simulink model "MAIN_simulation"  (R2021b)
settings: Solver=VariableStepAuto  StartTime=0.0  StopTime=10.0  RelTol=1e-3
values from neighbouring files (symbols this model uses):
  N = uint8(10)    [ParamSetup.m]
undefined symbols (not defined in the file or in its folder): Ankle, Hip, Knee, Left, Right, smiData, X, Y, Z
libraries: sm_lib x40, nesl_utility x15
(part 1 of 2)
settings Model: DataDictionary=ExoskeletonParameters.sldd  Creator=user  LastModifiedBy=khoi
settings SolverCC: AlgebraicLoopSolver=LineSearch
settings DebuggingCC: SFMachineParentedDataDiag=warning
settings ModelReferenceCC: EnableParallelModelReferenceBuilds=on  ModelReferenceMinAlgLoopOccurrences=on

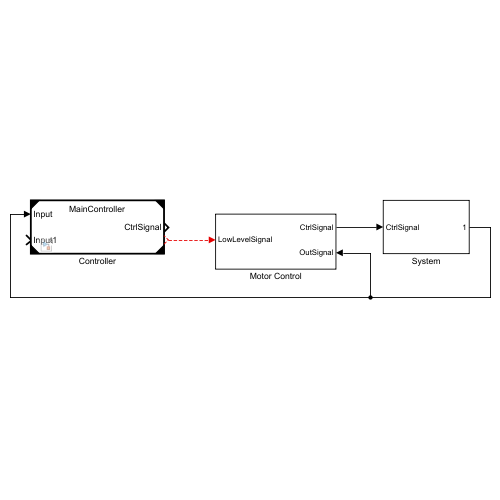
[thumbnail: Simulink's stored preview of the top-level diagram]
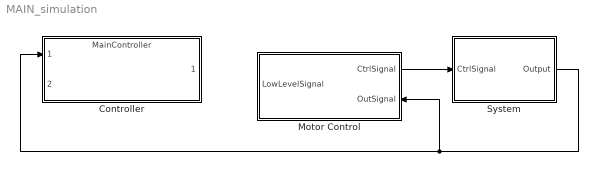
== system MAIN_simulation ==
  Controller : ModelReference  ModelNameDialog=MainController.slx  ModelReferenceVersion=1.32
  Motor Control : Subsystem
      settings: PortSchema="{\"entries\":[{\"content\":{\"sides\":[{\"content\":{\"connectorIds\":[\"In1\"]},\"type\":\"ConnectorPlacement.EquallySpacedRectSide\",\"uuid\":\"f726c4a5-dcc4-4232-8342-e270c8d2deba\"},{\"content\":{\"connectorIds\":[\"Out1\",\"In2\"],\"side\":\"RIGHT\"},\"type\":\"ConnectorPlacement.EquallySpacedRectSide\",\"uuid\":\"fdc8a78d-4edd-4abb-a00a-5ed0e9622b88\"},{\"content\":{\"connectorIds\":[],\"side\":\"TOP\"},\"type\":\"ConnectorPlacement.EquallySpacedRectSide\",\"uuid\":\"7577593d-02f9-4726-9a31-f3a7037643a8\"}]},\"type\":\"ConnectorPlacement.EquallySpacedConnector\",\"uuid\":\"d04c894f-3616-4ed1-83ff-a42822506ca7\"}],\"packageUris\":[\"http://schema.mathworks.com/mf0/Connector/19700101\"],\"version\":\"1.0\"}"
  System : Subsystem
  wires:
  System/1(Output) -> Controller/1, Motor Control/2(OutSignal)
  Motor Control/1(CtrlSignal) -> System/1(CtrlSignal)
  ? -> Motor Control/1(LowLevelSignal)

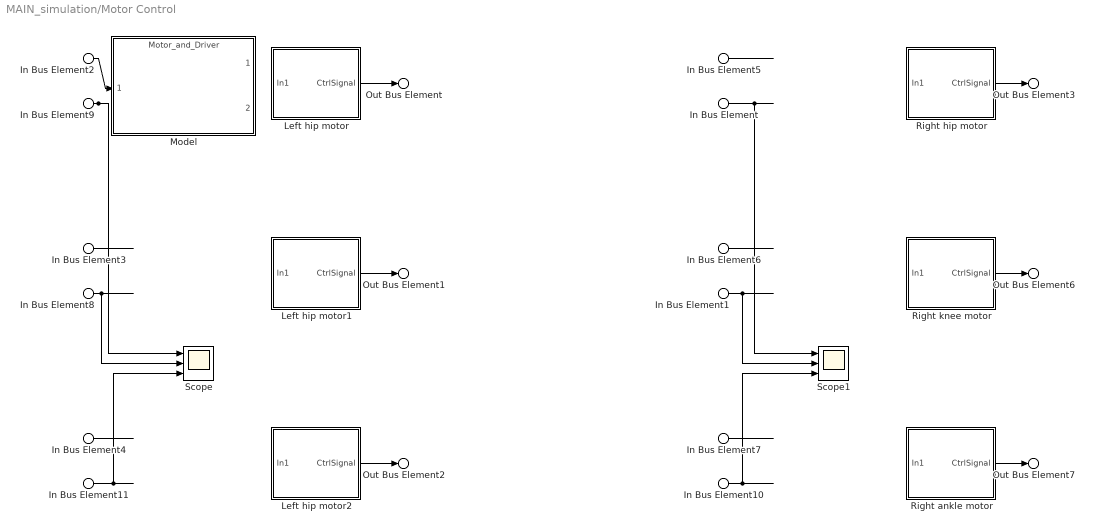
== system MAIN_simulation/Motor Control ==
  In Bus Element2 : Inport  PortName=LowLevelSignal  Element=Left.Hip.Angle
  In Bus Element3 : Inport  PortName=LowLevelSignal  Element=Left.Knee.Angle
  In Bus Element4 : Inport  PortName=LowLevelSignal  Element=Left.Ankle.Angle
  In Bus Element5 : Inport  PortName=LowLevelSignal  Element=Right.Hip.Angle
  In Bus Element6 : Inport  PortName=LowLevelSignal  Element=Right.Knee.Angle
  In Bus Element7 : Inport  PortName=LowLevelSignal  Element=Right.Ankle.Angle
  In Bus Element : Inport  Port=2  PortName=OutSignal  Element=Right.Hip.Angle
  In Bus Element1 : Inport  Port=2  PortName=OutSignal  Element=Right.Knee.Angle
  In Bus Element10 : Inport  Port=2  PortName=OutSignal  Element=Right.Ankle.Angle
  In Bus Element8 : Inport  Port=2  PortName=OutSignal  Element=Left.Knee.Angle
  In Bus Element9 : Inport  Port=2  PortName=OutSignal  Element=Left.Hip.Angle
  In Bus Element11 : Inport  Port=2  PortName=OutSignal  Element=Left.Ankle.Angle
  Left hip motor : Subsystem
  Left hip motor1 : Subsystem
  Left hip motor2 : Subsystem
  Model : ModelReference  ModelNameDialog=Motor_and_Driver.slx  ModelReferenceVersion=1.83
  Right ankle motor : Subsystem
  Right hip motor : Subsystem
  Right knee motor : Subsystem
  Scope : Scope  NumInputPorts=3
  Scope1 : Scope  NumInputPorts=3
  Out Bus Element : Outport  PortName=CtrlSignal  Element=Left.Hip
  Out Bus Element1 : Outport  PortName=CtrlSignal  Element=Left.Knee
  Out Bus Element2 : Outport  PortName=CtrlSignal  Element=Left.Ankle
  Out Bus Element3 : Outport  PortName=CtrlSignal  Element=Right.Hip
  Out Bus Element6 : Outport  PortName=CtrlSignal  Element=Right.Knee
  Out Bus Element7 : Outport  PortName=CtrlSignal  Element=Right.Ankle
  wires:
  Left hip motor/1(CtrlSignal) -> Out Bus Element/1
  ? -> Left hip motor/1(In1)
  In Bus Element9/1 -> Scope/1
  In Bus Element2/1 -> Model/1
  In Bus Element3/1 -> ?
  In Bus Element8/1 -> Scope/2
  ? -> Left hip motor1/1(In1)
  Left hip motor1/1(CtrlSignal) -> Out Bus Element1/1
  Left hip motor2/1(CtrlSignal) -> Out Bus Element2/1
  ? -> Left hip motor2/1(In1)
  In Bus Element11/1 -> Scope/3
  In Bus Element4/1 -> ?
  In Bus Element5/1 -> ?
  In Bus Element/1 -> Scope1/1
  ? -> Right hip motor/1(In1)
  Right hip motor/1(CtrlSignal) -> Out Bus Element3/1
  Right knee motor/1(CtrlSignal) -> Out Bus Element6/1
  ? -> Right knee motor/1(In1)
  In Bus Element1/1 -> Scope1/2
  In Bus Element6/1 -> ?
  In Bus Element7/1 -> ?
  In Bus Element10/1 -> Scope1/3
  Right ankle motor/1(CtrlSignal) -> Out Bus Element7/1
  ? -> Right ankle motor/1(In1)

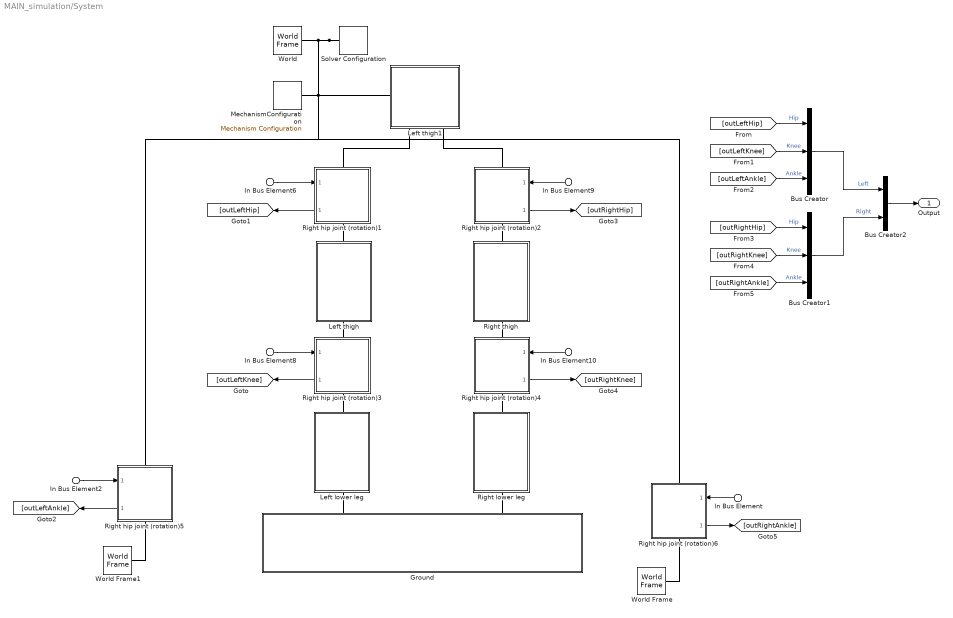
== system MAIN_simulation/System ==
  In Bus Element6 : Inport  PortName=CtrlSignal  Element=Left.Hip
  In Bus Element8 : Inport  PortName=CtrlSignal  Element=Left.Knee
  In Bus Element2 : Inport  PortName=CtrlSignal  Element=Left.Ankle
  In Bus Element9 : Inport  PortName=CtrlSignal  Element=Right.Hip
  In Bus Element10 : Inport  PortName=CtrlSignal  Element=Right.Knee
  In Bus Element : Inport  PortName=CtrlSignal  Element=Right.Ankle
  Bus Creator : BusCreator  Inputs=Hip,Knee,Ankle  OutDataTypeStr=Bus: LegSignal  NonVirtualBus=on
  Bus Creator1 : BusCreator  Inputs=Hip,Knee,Ankle  OutDataTypeStr=Bus: LegSignal  NonVirtualBus=on
  Bus Creator2 : BusCreator  Inputs=Left,Right  OutDataTypeStr=Bus: ExoskeletonSignal  NonVirtualBus=on
  Ground : Subsystem
      settings: PortSchema="{\"entries\":[{\"content\":{\"sides\":[{\"content\":{\"connectorIds\":[]},\"type\":\"ConnectorPlacement.EquallySpacedRectSide\",\"uuid\":\"bc708d77-af96-4d7d-95d3-fabc1bd4bef7\"},{\"content\":{\"connectorIds\":[],\"side\":\"RIGHT\"},\"type\":\"ConnectorPlacement.EquallySpacedRectSide\",\"uuid\":\"7d1ae7bb-4546-48a9-ac0a-f29757694b75\"},{\"content\":{\"connectorIds\":[\"LConn1\",\"LConn2\"],\"side\":\"TOP\"},\"type\":\"ConnectorPlacement.EquallySpacedRectSide\",\"uuid\":\"bbd1d651-6f83-40fc-b207-b59cdd7c8eb2\"}]},\"type\":\"ConnectorPlacement.EquallySpacedConnector\",\"uuid\":\"fc2fe8ec-6acb-4b8e-88eb-86a11b884530\"}],\"packageUris\":[\"http://schema.mathworks.com/mf0/Connector/19700101\"],\"version\":\"1.0\"}"
      mask Display: disp('Ground')
  Left lower leg : Subsystem
      settings: PortSchema="{\"entries\":[{\"content\":{\"sides\":[{\"content\":{\"connectorIds\":[]},\"type\":\"ConnectorPlacement.EquallySpacedRectSide\",\"uuid\":\"bc708d77-af96-4d7d-95d3-fabc1bd4bef7\"},{\"content\":{\"connectorIds\":[],\"side\":\"RIGHT\"},\"type\":\"ConnectorPlacement.EquallySpacedRectSide\",\"uuid\":\"7d1ae7bb-4546-48a9-ac0a-f29757694b75\"},{\"content\":{\"connectorIds\":[\"LConn1\"],\"side\":\"TOP\"},\"type\":\"ConnectorPlacement.EquallySpacedRectSide\",\"uuid\":\"bbd1d651-6f83-40fc-b207-b59cdd7c8eb2\"},{\"content\":{\"connectorIds\":[\"RConn1\"],\"side\":\"BOTTOM\"},\"type\":\"ConnectorPlacement.EquallySpacedRectSide\",\"uuid\":\"a7800cbb-99c0-4edf-9807-b8adb3def8d2\"}]},\"type\":\"ConnectorPlacement.EquallySpacedConnector\",\"uuid\":\"fc2fe8ec-6acb-4b8e-88eb-86a11b884530\"}],\"packageUris\":[\"http://schema.mathworks.com/mf0/Connector/19700101\"],\"version\":\"1.0\"}"
      mask Display: disp('Left lower leg')
  Left thigh : Subsystem
      settings: PortSchema="{\"entries\":[{\"content\":{\"sides\":[{\"content\":{\"connectorIds\":[]},\"type\":\"ConnectorPlacement.EquallySpacedRectSide\",\"uuid\":\"c448759e-36af-449c-acc8-d1dd18743b6b\"},{\"content\":{\"connectorIds\":[],\"side\":\"RIGHT\"},\"type\":\"ConnectorPlacement.EquallySpacedRectSide\",\"uuid\":\"f07dc0c7-5eca-4df9-b2f8-2f27b200d8d0\"},{\"content\":{\"connectorIds\":[\"LConn1\"],\"side\":\"TOP\"},\"type\":\"ConnectorPlacement.EquallySpacedRectSide\",\"uuid\":\"631955a4-1984-42ba-8529-31d94b2b0ecd\"},{\"content\":{\"connectorIds\":[\"RConn1\"],\"side\":\"BOTTOM\"},\"type\":\"ConnectorPlacement.EquallySpacedRectSide\",\"uuid\":\"95d177f4-b40a-41eb-aba2-65f8bb3c67f5\"}]},\"type\":\"ConnectorPlacement.EquallySpacedConnector\",\"uuid\":\"5d2bf2ac-7c34-4aa3-bc5b-7e42019ce5c4\"}],\"packageUris\":[\"http://schema.mathworks.com/mf0/Connector/19700101\"],\"version\":\"1.0\"}"
      mask Display: disp('Left upper leg')
  Left thigh1 : Subsystem
      settings: PortSchema="{\"entries\":[{\"content\":{\"sides\":[{\"content\":{\"connectorIds\":[\"LConn1\"]},\"type\":\"ConnectorPlacement.EquallySpacedRectSide\",\"uuid\":\"a4525506-eda0-44ad-aa11-265f693e0b1e\"},{\"content\":{\"connectorIds\":[],\"side\":\"RIGHT\"},\"type\":\"ConnectorPlacement.EquallySpacedRectSide\",\"uuid\":\"56f17016-b557-4494-9b64-34586218bf85\"},{\"content\":{\"connectorIds\":[\"LConn2\",\"LConn3\"],\"side\":\"TOP\"},\"type\":\"ConnectorPlacement.EquallySpacedRectSide\",\"uuid\":\"387d925d-8e4d-45ac-8af1-278822296279\"}]},\"type\":\"ConnectorPlacement.EquallySpacedConnector\",\"uuid\":\"2e8c75fc-9294-449c-97a7-b2eb1680b9f4\"}],\"packageUris\":[\"http://schema.mathworks.com/mf0/Connector/19700101\"],\"version\":\"1.0\"}"
      mask Display: disp('Slider')
  MechanismConfiguration : sm_lib/Utilities/Mechanism Configuration  UniformGravity=Constant  GravityVector=[0 0 -9.80665]  GravityUnits=m/s^2  LinearizationDelta=0.001  JointModeTransitionNonlinearIterations=2
  Right hip joint (rotation){1..6} (6 alike) : Subsystem  TreatAsAtomicUnit=on  ReferencedSubsystem=JointRotation
      settings: PortSchema="{\"entries\":[{\"content\":{\"sides\":[{\"content\":{\"connectorIds\":[\"In1\",\"Out1\"]},\"type\":\"ConnectorPlacement.EquallySpacedRectSide\",\"uuid\":\"c448759e-36af-449c-acc8-d1dd18743b6b\"},{\"content\":{\"connectorIds\":[],\"side\":\"RIGHT\"},\"type\":\"ConnectorPlacement.EquallySpacedRectSide\",\"uuid\":\"f07dc0c7-5eca-4df9-b2f8-2f27b200d8d0\"},{\"content\":{\"connectorIds\":[\"LConn1\"],\"side\":\"TOP\"},\"type\":\"ConnectorPlacement.EquallySpacedRectSide\",\"uuid\":\"631955a4-1984-42ba-8529-31d94b2b0ecd\"},{\"content\":{\"connectorIds\":[\"RConn1\"],\"side\":\"BOTTOM\"},\"type\":\"ConnectorPlacement.EquallySpacedRectSide\",\"uuid\":\"95d177f4-b40a-41eb-aba2-65f8bb3c67f5\"}]},\"type\":\"ConnectorPlacement.EquallySpacedConnector\",\"uuid\":\"5d2bf2ac-7c34-4aa3-bc5b-7e42019ce5c4\"}],\"packageUris\":[\"http://schema.mathworks.com/mf0/Connector/R2020b\"],\"version\":\"1.0\"}"
  Right lower leg : Subsystem
      settings: PortSchema="{\"entries\":[{\"content\":{\"sides\":[{\"content\":{\"connectorIds\":[]},\"type\":\"ConnectorPlacement.EquallySpacedRectSide\",\"uuid\":\"a018de65-cb0a-4a5a-a5af-2172e9083110\"},{\"content\":{\"connectorIds\":[],\"side\":\"RIGHT\"},\"type\":\"ConnectorPlacement.EquallySpacedRectSide\",\"uuid\":\"8c4c2bff-3dc0-4e7c-b633-b10883c57c05\"},{\"content\":{\"connectorIds\":[\"LConn1\"],\"side\":\"TOP\"},\"type\":\"ConnectorPlacement.EquallySpacedRectSide\",\"uuid\":\"6390764f-1055-472c-ada4-bb52f8a9a3b3\"},{\"content\":{\"connectorIds\":[\"RConn1\"],\"side\":\"BOTTOM\"},\"type\":\"ConnectorPlacement.EquallySpacedRectSide\",\"uuid\":\"97543a7b-2a12-40aa-8c09-035d5a148032\"}]},\"type\":\"ConnectorPlacement.EquallySpacedConnector\",\"uuid\":\"f5fe51f0-fa6d-49f2-bc30-0a046b03e837\"}],\"packageUris\":[\"http://schema.mathworks.com/mf0/Connector/19700101\"],\"version\":\"1.0\"}"
      mask Display: disp('Right lower leg')
  Right thigh : Subsystem
      settings: PortSchema="{\"entries\":[{\"content\":{\"sides\":[{\"content\":{\"connectorIds\":[]},\"type\":\"ConnectorPlacement.EquallySpacedRectSide\",\"uuid\":\"bc708d77-af96-4d7d-95d3-fabc1bd4bef7\"},{\"content\":{\"connectorIds\":[],\"side\":\"RIGHT\"},\"type\":\"ConnectorPlacement.EquallySpacedRectSide\",\"uuid\":\"7d1ae7bb-4546-48a9-ac0a-f29757694b75\"},{\"content\":{\"connectorIds\":[\"LConn1\"],\"side\":\"TOP\"},\"type\":\"ConnectorPlacement.EquallySpacedRectSide\",\"uuid\":\"bbd1d651-6f83-40fc-b207-b59cdd7c8eb2\"},{\"content\":{\"connectorIds\":[\"RConn1\"],\"side\":\"BOTTOM\"},\"type\":\"ConnectorPlacement.EquallySpacedRectSide\",\"uuid\":\"f402502e-27b9-4bf6-8618-1cf773e950eb\"}]},\"type\":\"ConnectorPlacement.EquallySpacedConnector\",\"uuid\":\"fc2fe8ec-6acb-4b8e-88eb-86a11b884530\"}],\"packageUris\":[\"http://schema.mathworks.com/mf0/Connector/19700101\"],\"version\":\"1.0\"}"
      mask Display: disp('Right upper leg')
  Solver Configuration : nesl_utility/Solver Configuration  PhysicalDomain=network_engine_domain  SubClassName=solver  LeftPortType=input  RightPortType=generic  Tones=[]  Harmonics=[]  SimulateNoise=off  Profile=off  UseLocalSampling=off  EnableSwitchedLinearOptims=on  FrequencyDomain=off  UseCCode=off  RelTol=0.001  AbsTol=1e-06  MinStep=1e-09  ToWorkspace=off  RevertToSquareIcSolve=off  NumHomotopyIterations=100  PhasorMode=off  PhasorModeNumHarmonics=1  DoDC=off  ResidualTolerance=1e-09  UseLocalSolver=off  LocalSolverChoice=NE_BACKWARD_EULER_ADVANCER  LocalSolverSampleTime=0.001  DoFixedCost=off  MaxNonlinIter=3  MaxModeIter=2  ComputeImpulses=off  ImpulseIterations=2  LinearAlgebra=Sparse  EquationFormulation=NE_TIME_EF  DelaysMemoryBudget=1024  AutomaticFiltering=on  FilteringTimeConstant=0.001  PartitionStorageMethod=AS_NEEDED  PartitionMemoryBudget=1024  PartitionMethod=FAST
      settings: SourceProductBaseCode=PW,SS
  World : sm_lib/Frames and Transforms/World Frame
  World Frame : sm_lib/Frames and Transforms/World Frame
  World Frame1 : sm_lib/Frames and Transforms/World Frame
  Output : Outport
  wires:
  In Bus Element6/1 -> Right hip joint (rotation)1/1
  In Bus Element8/1 -> Right hip joint (rotation)3/1
  In Bus Element9/1 -> Right hip joint (rotation)2/1
  In Bus Element10/1 -> Right hip joint (rotation)4/1
  Right hip joint (rotation)2/1 -> [outRightHip]
  Right hip joint (rotation)4/1 -> [outRightKnee]
  Right hip joint (rotation)3/1 -> [outLeftKnee]
  Right hip joint (rotation)1/1 -> [outLeftHip]
  Right hip joint (rotation)6/1 -> [outRightAnkle]
  In Bus Element/1 -> Right hip joint (rotation)6/1
  Right hip joint (rotation)5/1 -> [outLeftAnkle]
  In Bus Element2/1 -> Right hip joint (rotation)5/1
  [outLeftHip] -> Bus Creator/1  "Hip"
  [outLeftKnee] -> Bus Creator/2  "Knee"
  [outLeftAnkle] -> Bus Creator/3  "Ankle"
  [outRightHip] -> Bus Creator1/1  "Hip"
  [outRightKnee] -> Bus Creator1/2  "Knee"
  [outRightAnkle] -> Bus Creator1/3  "Ankle"
  Bus Creator/1 -> Bus Creator2/1  "Left"
  Bus Creator1/1 -> Bus Creator2/2  "Right"
  Bus Creator2/1 -> Output/1
  connections:
  Right hip joint (rotation)1/RConn1 -- Left thigh/LConn1
  Right hip joint (rotation)3/LConn1 -- Left thigh/RConn1
  Right hip joint (rotation)2/RConn1 -- Right thigh/LConn1
  Right hip joint (rotation)4/LConn1 -- Right thigh/RConn1
  Right hip joint (rotation)3/RConn1 -- Left lower leg/LConn1
  Right hip joint (rotation)4/RConn1 -- Right lower leg/LConn1
  Right lower leg/RConn1 -- Ground/LConn2
  Ground/LConn1 -- Left lower leg/RConn1
  Right hip joint (rotation)2/LConn1 -- Left thigh1/LConn3
  Right hip joint (rotation)1/LConn1 -- Left thigh1/LConn2
  Solver Configuration/RConn1 -- Right hip joint (rotation)5/LConn1 -- Right hip joint (rotation)6/LConn1 -- Left thigh1/LConn1 -- MechanismConfiguration/RConn1 -- World/RConn1
  Right hip joint (rotation)6/RConn1 -- World Frame/RConn1
  World Frame1/RConn1 -- Right hip joint (rotation)5/RConn1

== system MAIN_simulation/Motor Control/Left hip motor ==
  In1 : Inport
  Bus Selector : BusSelector  OutputSignals=angle,speed,torque
  Model : ModelReference  ModelNameDialog=Motor.slx  ModelReferenceVersion=1.10
  Out Bus Element : Outport  PortName=CtrlSignal  Element=Angle
  Out Bus Element2 : Outport  PortName=CtrlSignal  Element=Speed
  Out Bus Element3 : Outport  PortName=CtrlSignal  Element=Torque
  wires:
  Bus Selector/1 -> Out Bus Element/1  "<angle>"
  Bus Selector/3 -> Out Bus Element3/1  "<torque>"
  Bus Selector/2 -> Out Bus Element2/1  "<speed>"
  In1/1 -> Model/1
  Model/1 -> Bus Selector/1

== system MAIN_simulation/Motor Control/Left hip motor1 ==
  In1 : Inport
  Bus Selector : BusSelector  OutputSignals=angle,speed,torque
  Model : ModelReference  ModelNameDialog=Motor.slx  ModelReferenceVersion=1.10
  Out Bus Element : Outport  PortName=CtrlSignal  Element=Angle
  Out Bus Element2 : Outport  PortName=CtrlSignal  Element=Speed
  Out Bus Element3 : Outport  PortName=CtrlSignal  Element=Torque
  wires:
  Model/1 -> Bus Selector/1
  In1/1 -> Model/1
  Bus Selector/2 -> Out Bus Element2/1  "<speed>"
  Bus Selector/3 -> Out Bus Element3/1  "<torque>"
  Bus Selector/1 -> Out Bus Element/1  "<angle>"

== system MAIN_simulation/Motor Control/Left hip motor2 ==
  In1 : Inport
  Bus Selector : BusSelector  OutputSignals=angle,speed,torque
  Model : ModelReference  ModelNameDialog=Motor.slx  ModelReferenceVersion=1.10
  Out Bus Element : Outport  PortName=CtrlSignal  Element=Angle
  Out Bus Element2 : Outport  PortName=CtrlSignal  Element=Speed
  Out Bus Element3 : Outport  PortName=CtrlSignal  Element=Torque
  wires:
  Bus Selector/1 -> Out Bus Element/1  "<angle>"
  Bus Selector/3 -> Out Bus Element3/1  "<torque>"
  Bus Selector/2 -> Out Bus Element2/1  "<speed>"
  In1/1 -> Model/1
  Model/1 -> Bus Selector/1

== system MAIN_simulation/Motor Control/Right ankle motor ==
  In1 : Inport
  Bus Selector : BusSelector  OutputSignals=angle,speed,torque
  Model : ModelReference  ModelNameDialog=Motor.slx  ModelReferenceVersion=1.10
  Out Bus Element : Outport  PortName=CtrlSignal  Element=Angle
  Out Bus Element2 : Outport  PortName=CtrlSignal  Element=Speed
  Out Bus Element3 : Outport  PortName=CtrlSignal  Element=Torque
  wires:
  Model/1 -> Bus Selector/1
  In1/1 -> Model/1
  Bus Selector/2 -> Out Bus Element2/1  "<speed>"
  Bus Selector/3 -> Out Bus Element3/1  "<torque>"
  Bus Selector/1 -> Out Bus Element/1  "<angle>"

== system MAIN_simulation/Motor Control/Right hip motor ==
  In1 : Inport
  Bus Selector : BusSelector  OutputSignals=angle,speed,torque
  Model : ModelReference  ModelNameDialog=Motor.slx  ModelReferenceVersion=1.10
  Out Bus Element : Outport  PortName=CtrlSignal  Element=Angle
  Out Bus Element2 : Outport  PortName=CtrlSignal  Element=Speed
  Out Bus Element3 : Outport  PortName=CtrlSignal  Element=Torque
  wires:
  Model/1 -> Bus Selector/1
  In1/1 -> Model/1
  Bus Selector/2 -> Out Bus Element2/1  "<speed>"
  Bus Selector/3 -> Out Bus Element3/1  "<torque>"
  Bus Selector/1 -> Out Bus Element/1  "<angle>"

== system MAIN_simulation/Motor Control/Right knee motor ==
  In1 : Inport
  Bus Selector : BusSelector  OutputSignals=angle,speed,torque
  Model : ModelReference  ModelNameDialog=Motor.slx  ModelReferenceVersion=1.10
  Out Bus Element : Outport  PortName=CtrlSignal  Element=Angle
  Out Bus Element2 : Outport  PortName=CtrlSignal  Element=Speed
  Out Bus Element3 : Outport  PortName=CtrlSignal  Element=Torque
  wires:
  Bus Selector/1 -> Out Bus Element/1  "<angle>"
  Bus Selector/3 -> Out Bus Element3/1  "<torque>"
  Bus Selector/2 -> Out Bus Element2/1  "<speed>"
  In1/1 -> Model/1
  Model/1 -> Bus Selector/1

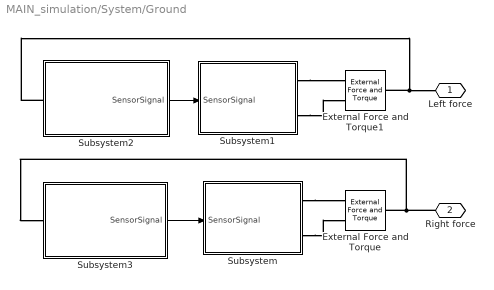
== system MAIN_simulation/System/Ground ==
  External Force and Torque : sm_lib/Forces and Torques/External Force and Torque  ForceResolutionFrame=World  EnableForceX=on  EnableForceY=off  EnableForceZ=on  EnableForce=off  TorqueResolutionFrame=AttachedFrame  EnableTorqueX=off  EnableTorqueY=off  EnableTorqueZ=off  EnableTorque=off
  External Force and Torque1 : sm_lib/Forces and Torques/External Force and Torque  ForceResolutionFrame=World  EnableForceX=on  EnableForceY=off  EnableForceZ=on  EnableForce=off  TorqueResolutionFrame=AttachedFrame  EnableTorqueX=off  EnableTorqueY=off  EnableTorqueZ=off  EnableTorque=off
  Subsystem : Subsystem
  Subsystem1 : Subsystem
  Subsystem2 : Subsystem
      settings: PortSchema="{\"entries\":[{\"content\":{\"sides\":[{\"content\":{\"connectorIds\":[\"Out1\"]},\"type\":\"ConnectorPlacement.EquallySpacedRectSide\",\"uuid\":\"864ab75a-2756-43ae-b944-4374333ccbae\"},{\"content\":{\"connectorIds\":[\"RConn1\"],\"side\":\"RIGHT\"},\"type\":\"ConnectorPlacement.EquallySpacedRectSide\",\"uuid\":\"2e2c1796-3401-45b1-983f-ef4384911bb4\"},{\"content\":{\"connectorIds\":[],\"side\":\"TOP\"},\"type\":\"ConnectorPlacement.EquallySpacedRectSide\",\"uuid\":\"e5b055f7-3a4b-4796-9b7c-66816c07d052\"}]},\"type\":\"ConnectorPlacement.EquallySpacedConnector\",\"uuid\":\"da74978d-57f5-49a8-97e6-4c6dbca8bf40\"}],\"packageUris\":[\"http://schema.mathworks.com/mf0/Connector/19700101\"],\"version\":\"1.0\"}"
  Subsystem3 : Subsystem
  Left force : PMIOPort  Side=Left
  Right force : PMIOPort  Port=2  Side=Left
  wires:
  Subsystem3/1(SensorSignal) -> Subsystem/1(SensorSignal)
  Subsystem2/1(SensorSignal) -> Subsystem1/1(SensorSignal)
  connections:
  Subsystem/RConn1 -- External Force and Torque/LConn1
  Subsystem1/RConn1 -- External Force and Torque1/LConn1
  Subsystem2/RConn1 -- Left force/RConn1 -- External Force and Torque1/RConn1
  Subsystem/RConn2 -- External Force and Torque/LConn2
  Subsystem1/RConn2 -- External Force and Torque1/LConn2
  Right force/RConn1 -- External Force and Torque/RConn1 -- Subsystem3/LConn1

== system MAIN_simulation/System/Left lower leg ==
  ReferenceFrame : sm_lib/Frames and Transforms/Reference Frame
  Solid : sm_lib/Body Elements/File Solid  ExtGeomFileName=Part4_Left_Default_sldprt.STEP  UnitType=FromFile  ExtGeomFileUnits=m  StepReaderType=HEX  ExportConvexHullGeometry=off  InertiaType=Custom  Mass=10  MassUnits=kg  CenterOfMass=[0 0 0]  CenterOfMassUnits=mm  MomentsOfInertia=[0 0 0]  MomentsOfInertiaUnits=kg*mm^2  ProductsOfInertia=[0 0 0]  ProductsOfInertiaUnits=kg*mm^2  BasedOnType=Density  Density=1000  DensityUnits=kg/m^3  DoExposeReferenceFrame=on  SerializedFrames=<Frames/>  GraphicType=FromGeometry  MarkerShape=Sphere  MarkerSize=10  GraphicVisPropType=SimpleVisualProperties  GraphicDiffuseColor=smiData.Solid(7).color  GraphicSpecularColor=[0.5 0.5 0.5 1.0]  GraphicAmbientColor=[0.15 0.15 0.15 1.0]  GraphicEmissiveColor=[0.0 0.0 0.0 1.0]  GraphicShininess=75  GraphicOpacity=smiData.Solid(7).opacity
  Transform : sm_lib/Frames and Transforms/Rigid Transform  TranslationMethod=Cartesian  TranslationStandardOffset=0  TranslationLengthUnit=mm  TranslationStandardAxis=+Z  TranslationCartesianOffset=smiData.RigidTransform(6).translation  TranslationROffset=0  TranslationROffsetUnits=m  TranslationZOffset=0  TranslationZOffsetUnits=m  TranslationThetaOffset=0  TranslationThetaOffsetUnits=deg  RotationMethod=ArbitraryAxis  RotationAngleUnits=rad  RotationStandardAxis=+Z  RotationAngle=smiData.RigidTransform(6).angle  RotationArbitraryAxis=smiData.RigidTransform(6).axis  FollAlignAxisA=+X  BaseAlignAxisA=+Y  FollAlignAxisB=+Y  BaseAlignAxisB=+Z  RotationSequenceAxes=FollowerAxes  RotationSequence=XYX  RotationSequenceAngles=[0 0 0]  RotationSequenceAnglesUnits=deg  RotationMatrix=[1 0 0; 0 1 0; 0 0 1]
  From knee joint : PMIOPort  Side=Left
  "To ground " : PMIOPort  Port=2  Side=Right
  connections:
  ReferenceFrame/RConn1 -- "To ground "/RConn1 -- Transform/LConn1 -- Solid/RConn1
  From knee joint/RConn1 -- Transform/RConn1

== system MAIN_simulation/System/Left thigh ==
  ReferenceFrame : sm_lib/Frames and Transforms/Reference Frame
  Solid : sm_lib/Body Elements/File Solid  ExtGeomFileName=Part3_Left_Default_sldprt.STEP  UnitType=FromFile  ExtGeomFileUnits=m  StepReaderType=HEX  ExportConvexHullGeometry=off  InertiaType=Custom  Mass=10  MassUnits=kg  CenterOfMass=[0 0 0]  CenterOfMassUnits=mm  MomentsOfInertia=[0 0 0]  MomentsOfInertiaUnits=kg*mm^2  ProductsOfInertia=[0 0 0]  ProductsOfInertiaUnits=kg*mm^2  BasedOnType=Density  Density=1000  DensityUnits=kg/m^3  DoExposeReferenceFrame=on  SerializedFrames=<Frames/>  GraphicType=FromGeometry  MarkerShape=Sphere  MarkerSize=10  GraphicVisPropType=SimpleVisualProperties  GraphicDiffuseColor=smiData.Solid(2).color  GraphicSpecularColor=[0.5 0.5 0.5 1.0]  GraphicAmbientColor=[0.15 0.15 0.15 1.0]  GraphicEmissiveColor=[0.0 0.0 0.0 1.0]  GraphicShininess=75  GraphicOpacity=smiData.Solid(2).opacity
  Transform : sm_lib/Frames and Transforms/Rigid Transform  TranslationMethod=Cartesian  TranslationStandardOffset=0  TranslationLengthUnit=mm  TranslationStandardAxis=+Z  TranslationCartesianOffset=smiData.RigidTransform(5).translation  TranslationROffset=0  TranslationROffsetUnits=m  TranslationZOffset=0  TranslationZOffsetUnits=m  TranslationThetaOffset=0  TranslationThetaOffsetUnits=deg  RotationMethod=ArbitraryAxis  RotationAngleUnits=rad  RotationStandardAxis=+Z  RotationAngle=smiData.RigidTransform(5).angle  RotationArbitraryAxis=smiData.RigidTransform(5).axis  FollAlignAxisA=+X  BaseAlignAxisA=+Y  FollAlignAxisB=+Y  BaseAlignAxisB=+Z  RotationSequenceAxes=FollowerAxes  RotationSequence=XYX  RotationSequenceAngles=[0 0 0]  RotationSequenceAnglesUnits=deg  RotationMatrix=[1 0 0; 0 1 0; 0 0 1]
  Transform1 : sm_lib/Frames and Transforms/Rigid Transform  TranslationMethod=Cartesian  TranslationStandardOffset=0  TranslationLengthUnit=mm  TranslationStandardAxis=+Z  TranslationCartesianOffset=smiData.RigidTransform(14).translation  TranslationROffset=0  TranslationROffsetUnits=m  TranslationZOffset=0  TranslationZOffsetUnits=m  TranslationThetaOffset=0  TranslationThetaOffsetUnits=deg  RotationMethod=ArbitraryAxis  RotationAngleUnits=rad  RotationStandardAxis=+Z  RotationAngle=smiData.RigidTransform(14).angle  RotationArbitraryAxis=smiData.RigidTransform(14).axis  FollAlignAxisA=+X  BaseAlignAxisA=+Y  FollAlignAxisB=+Y  BaseAlignAxisB=+Z  RotationSequenceAxes=FollowerAxes  RotationSequence=XYX  RotationSequenceAngles=[0 0 0]  RotationSequenceAnglesUnits=deg  RotationMatrix=[1 0 0; 0 1 0; 0 0 1]
  From hip joint : PMIOPort  Side=Left
  To knee joint : PMIOPort  Port=2  Side=Right
  connections:
  Transform1/LConn1 -- ReferenceFrame/RConn1 -- Transform/LConn1 -- Solid/RConn1
  Transform1/RConn1 -- From hip joint/RConn1
  Transform/RConn1 -- To knee joint/RConn1

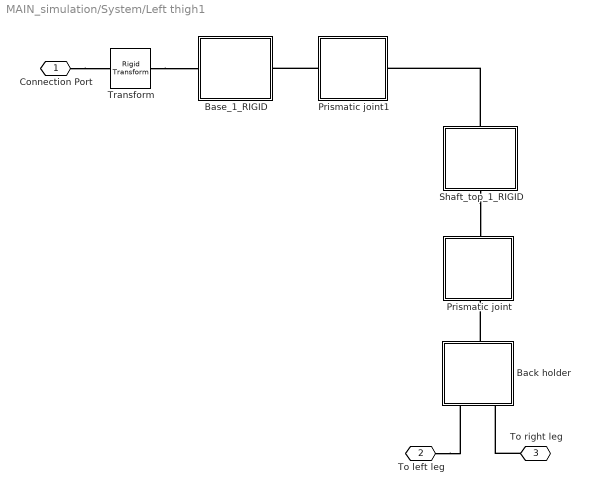
== system MAIN_simulation/System/Left thigh1 ==
  Back holder : Subsystem
      mask Display: disp('Back holder')
  Base_1_RIGID : Subsystem
      mask Display: disp('Horizontal\nslider')
  Prismatic joint : Subsystem
      settings: PortSchema="{\"entries\":[{\"content\":{\"sides\":[{\"content\":{\"connectorIds\":[]},\"type\":\"ConnectorPlacement.EquallySpacedRectSide\",\"uuid\":\"7c9e08f6-9071-42d8-9121-ca11c796013d\"},{\"content\":{\"connectorIds\":[],\"side\":\"RIGHT\"},\"type\":\"ConnectorPlacement.EquallySpacedRectSide\",\"uuid\":\"acead171-32e9-4018-ae0e-b918e8867532\"},{\"content\":{\"connectorIds\":[\"LConn1\"],\"side\":\"TOP\"},\"type\":\"ConnectorPlacement.EquallySpacedRectSide\",\"uuid\":\"203dcc15-0bf7-4902-9664-1d3a003d7f5c\"},{\"content\":{\"connectorIds\":[\"RConn1\"],\"side\":\"BOTTOM\"},\"type\":\"ConnectorPlacement.EquallySpacedRectSide\",\"uuid\":\"6a6e625a-c533-4c2d-aa18-e243746d71b6\"}]},\"type\":\"ConnectorPlacement.EquallySpacedConnector\",\"uuid\":\"3a60191e-8ae5-4bd7-925e-02d87dcf7b01\"}],\"packageUris\":[\"http://schema.mathworks.com/mf0/Connector/19700101\"],\"version\":\"1.0\"}"
      mask Display: disp('Prismatic\njoint')
  Prismatic joint1 : Subsystem
      mask Display: disp('Prismatic\njoint')
  Shaft_top_1_RIGID : Subsystem
      settings: PortSchema="{\"entries\":[{\"content\":{\"sides\":[{\"content\":{\"connectorIds\":[]},\"type\":\"ConnectorPlacement.EquallySpacedRectSide\",\"uuid\":\"a4525506-eda0-44ad-aa11-265f693e0b1e\"},{\"content\":{\"connectorIds\":[],\"side\":\"RIGHT\"},\"type\":\"ConnectorPlacement.EquallySpacedRectSide\",\"uuid\":\"56f17016-b557-4494-9b64-34586218bf85\"},{\"content\":{\"connectorIds\":[\"LConn1\"],\"side\":\"TOP\"},\"type\":\"ConnectorPlacement.EquallySpacedRectSide\",\"uuid\":\"387d925d-8e4d-45ac-8af1-278822296279\"},{\"content\":{\"connectorIds\":[\"RConn1\"],\"side\":\"BOTTOM\"},\"type\":\"ConnectorPlacement.EquallySpacedRectSide\",\"uuid\":\"791f4cfe-d541-4881-9a96-44e48ab9d38d\"}]},\"type\":\"ConnectorPlacement.EquallySpacedConnector\",\"uuid\":\"2e8c75fc-9294-449c-97a7-b2eb1680b9f4\"}],\"packageUris\":[\"http://schema.mathworks.com/mf0/Connector/19700101\"],\"version\":\"1.0\"}"
      mask Display: disp('Vertical\nslider')
  Transform : sm_lib/Frames and Transforms/Rigid Transform  TranslationMethod=Cartesian  TranslationStandardOffset=0  TranslationLengthUnit=mm  TranslationStandardAxis=+Z  TranslationCartesianOffset=smiData.RigidTransform(4).translation  TranslationROffset=0  TranslationROffsetUnits=m  TranslationZOffset=0  TranslationZOffsetUnits=m  TranslationThetaOffset=0  TranslationThetaOffsetUnits=deg  RotationMethod=ArbitraryAxis  RotationAngleUnits=rad  RotationStandardAxis=+Z  RotationAngle=smiData.RigidTransform(4).angle  RotationArbitraryAxis=smiData.RigidTransform(4).axis  FollAlignAxisA=+X  BaseAlignAxisA=+Y  FollAlignAxisB=+Y  BaseAlignAxisB=+Z  RotationSequenceAxes=FollowerAxes  RotationSequence=XYX  RotationSequenceAngles=[0 0 0]  RotationSequenceAnglesUnits=deg  RotationMatrix=[1 0 0; 0 1 0; 0 0 1]
  Connection Port : PMIOPort  Side=Left
  To left leg : PMIOPort  Port=2  Side=Left
  To right leg : PMIOPort  Port=3  Side=Left
  connections:
  Transform/RConn1 -- Base_1_RIGID/LConn1
  Prismatic joint1/LConn1 -- Base_1_RIGID/RConn1
  Shaft_top_1_RIGID/LConn1 -- Prismatic joint1/RConn1
  Shaft_top_1_RIGID/RConn1 -- Prismatic joint/LConn1
  To left leg/RConn1 -- Back holder/RConn2
  To right leg/RConn1 -- Back holder/RConn1
  Back holder/LConn1 -- Prismatic joint/RConn1
  Connection Port/RConn1 -- Transform/LConn1

== system MAIN_simulation/System/Right lower leg ==
  ReferenceFrame : sm_lib/Frames and Transforms/Reference Frame
  Solid : sm_lib/Body Elements/File Solid  ExtGeomFileName=Part4_Right_Default_sldprt.STEP  UnitType=FromFile  ExtGeomFileUnits=m  StepReaderType=HEX  ExportConvexHullGeometry=off  InertiaType=Custom  Mass=10  MassUnits=kg  CenterOfMass=[0 0 0]  CenterOfMassUnits=mm  MomentsOfInertia=[0 0 0]  MomentsOfInertiaUnits=kg*mm^2  ProductsOfInertia=[0 0 0]  ProductsOfInertiaUnits=kg*mm^2  BasedOnType=Density  Density=1000  DensityUnits=kg/m^3  DoExposeReferenceFrame=on  SerializedFrames=<Frames/>  GraphicType=FromGeometry  MarkerShape=Sphere  MarkerSize=10  GraphicVisPropType=SimpleVisualProperties  GraphicDiffuseColor=smiData.Solid(1).color  GraphicSpecularColor=[0.5 0.5 0.5 1.0]  GraphicAmbientColor=[0.15 0.15 0.15 1.0]  GraphicEmissiveColor=[0.0 0.0 0.0 1.0]  GraphicShininess=75  GraphicOpacity=smiData.Solid(1).opacity
  Transform : sm_lib/Frames and Transforms/Rigid Transform  TranslationMethod=Cartesian  TranslationStandardOffset=0  TranslationLengthUnit=mm  TranslationStandardAxis=+Z  TranslationCartesianOffset=smiData.RigidTransform(8).translation  TranslationROffset=0  TranslationROffsetUnits=m  TranslationZOffset=0  TranslationZOffsetUnits=m  TranslationThetaOffset=0  TranslationThetaOffsetUnits=deg  RotationMethod=ArbitraryAxis  RotationAngleUnits=rad  RotationStandardAxis=+Z  RotationAngle=smiData.RigidTransform(8).angle  RotationArbitraryAxis=smiData.RigidTransform(8).axis  FollAlignAxisA=+X  BaseAlignAxisA=+Y  FollAlignAxisB=+Y  BaseAlignAxisB=+Z  RotationSequenceAxes=FollowerAxes  RotationSequence=XYX  RotationSequenceAngles=[0 0 0]  RotationSequenceAnglesUnits=deg  RotationMatrix=[1 0 0; 0 1 0; 0 0 1]
  From knee joint : PMIOPort  Side=Left
  To ground : PMIOPort  Port=2  Side=Right
  connections:
  From knee joint/RConn1 -- Transform/RConn1
  Transform/LConn1 -- ReferenceFrame/RConn1 -- Solid/RConn1 -- To ground/RConn1

== system MAIN_simulation/System/Right thigh ==
  ReferenceFrame : sm_lib/Frames and Transforms/Reference Frame
  Solid : sm_lib/Body Elements/File Solid  ExtGeomFileName=Part3_Right_Default_sldprt.STEP  UnitType=FromFile  ExtGeomFileUnits=m  StepReaderType=HEX  ExportConvexHullGeometry=off  InertiaType=Custom  Mass=10  MassUnits=kg  CenterOfMass=[0 0 0]  CenterOfMassUnits=mm  MomentsOfInertia=[0 0 0]  MomentsOfInertiaUnits=kg*mm^2  ProductsOfInertia=[0 0 0]  ProductsOfInertiaUnits=kg*mm^2  BasedOnType=Density  Density=1000  DensityUnits=kg/m^3  DoExposeReferenceFrame=on  SerializedFrames=<Frames/>  GraphicType=FromGeometry  MarkerShape=Sphere  MarkerSize=10  GraphicVisPropType=SimpleVisualProperties  GraphicDiffuseColor=smiData.Solid(4).color  GraphicSpecularColor=[0.5 0.5 0.5 1.0]  GraphicAmbientColor=[0.15 0.15 0.15 1.0]  GraphicEmissiveColor=[0.0 0.0 0.0 1.0]  GraphicShininess=75  GraphicOpacity=smiData.Solid(4).opacity
  Transform : sm_lib/Frames and Transforms/Rigid Transform  TranslationMethod=Cartesian  TranslationStandardOffset=0  TranslationLengthUnit=mm  TranslationStandardAxis=+Z  TranslationCartesianOffset=smiData.RigidTransform(7).translation  TranslationROffset=0  TranslationROffsetUnits=m  TranslationZOffset=0  TranslationZOffsetUnits=m  TranslationThetaOffset=0  TranslationThetaOffsetUnits=deg  RotationMethod=ArbitraryAxis  RotationAngleUnits=rad  RotationStandardAxis=+Z  RotationAngle=smiData.RigidTransform(7).angle  RotationArbitraryAxis=smiData.RigidTransform(7).axis  FollAlignAxisA=+X  BaseAlignAxisA=+Y  FollAlignAxisB=+Y  BaseAlignAxisB=+Z  RotationSequenceAxes=FollowerAxes  RotationSequence=XYX  RotationSequenceAngles=[0 0 0]  RotationSequenceAnglesUnits=deg  RotationMatrix=[1 0 0; 0 1 0; 0 0 1]
  Transform1 : sm_lib/Frames and Transforms/Rigid Transform  TranslationMethod=Cartesian  TranslationStandardOffset=0  TranslationLengthUnit=mm  TranslationStandardAxis=+Z  TranslationCartesianOffset=smiData.RigidTransform(10).translation  TranslationROffset=0  TranslationROffsetUnits=m  TranslationZOffset=0  TranslationZOffsetUnits=m  TranslationThetaOffset=0  TranslationThetaOffsetUnits=deg  RotationMethod=ArbitraryAxis  RotationAngleUnits=rad  RotationStandardAxis=+Z  RotationAngle=smiData.RigidTransform(10).angle  RotationArbitraryAxis=smiData.RigidTransform(10).axis  FollAlignAxisA=+X  BaseAlignAxisA=+Y  FollAlignAxisB=+Y  BaseAlignAxisB=+Z  RotationSequenceAxes=FollowerAxes  RotationSequence=XYX  RotationSequenceAngles=[0 0 0]  RotationSequenceAnglesUnits=deg  RotationMatrix=[1 0 0; 0 1 0; 0 0 1]
  From hip joint : PMIOPort  Side=Left
  To knee joint : PMIOPort  Port=2  Side=Right
  connections:
  Solid/RConn1 -- ReferenceFrame/RConn1 -- Transform/LConn1 -- Transform1/LConn1
  From hip joint/RConn1 -- Transform1/RConn1
  To knee joint/RConn1 -- Transform/RConn1

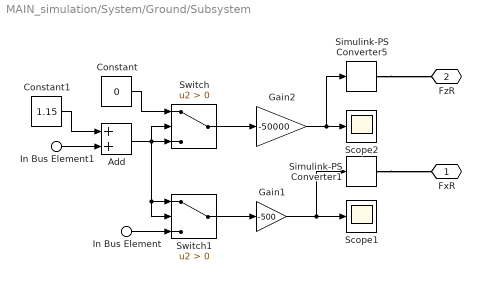
== system MAIN_simulation/System/Ground/Subsystem ==
  In Bus Element : Inport  PortName=SensorSignal  Element=Velocity.xAxis
  In Bus Element1 : Inport  PortName=SensorSignal  Element=Position.zAxis
  Add : Sum
  Constant : Constant  Value=0
  Constant1 : Constant  Value=1.15
  Gain1 : Gain  Gain=-500
  Gain2 : Gain  Gain=-50000
  Scope1 : Scope
  Scope2 : Scope
  Simulink-PS Converter1 : nesl_utility/Simulink-PS Converter  PhysicalDomain=network_engine_domain  SubClassName=ps_input  LeftPortType=input  RightPortType=output  PseudoPeriodic=off  Frequencies=[]  NoiseDistribution=none  NoiseParameters=[]  Unit=N  AffineConversion=off  FilteringAndDerivatives=filter  SimscapeFilterOrder=2  InputFilterTimeConstant=0.001  UdotUserProvided=0
      settings: SourceProductBaseCode=PW,SS
  Simulink-PS Converter5 : nesl_utility/Simulink-PS Converter  PhysicalDomain=network_engine_domain  SubClassName=ps_input  LeftPortType=input  RightPortType=output  PseudoPeriodic=off  Frequencies=[]  NoiseDistribution=none  NoiseParameters=[]  Unit=N  AffineConversion=off  FilteringAndDerivatives=filter  SimscapeFilterOrder=2  InputFilterTimeConstant=0.001  UdotUserProvided=0
      settings: SourceProductBaseCode=PW,SS
  Switch : Switch  Criteria=u2 > Threshold
  Switch1 : Switch  Criteria=u2 > Threshold
  FxR : PMIOPort  Side=Right
  FzR : PMIOPort  Port=2  Side=Right
  wires:
  Constant1/1 -> Add/1
  Gain1/1 -> Scope1/1, Simulink-PS Converter1/1
  In Bus Element/1 -> Switch1/3
  In Bus Element1/1 -> Add/2
  Constant/1 -> Switch/1
  Switch/1 -> Gain2/1
  Switch1/1 -> Gain1/1
  Gain2/1 -> Scope2/1, Simulink-PS Converter5/1
  Add/1 -> Switch1/1, Switch1/2, Switch/3, Switch/2
  connections:
  Simulink-PS Converter1/RConn1 -- FxR/RConn1
  Simulink-PS Converter5/RConn1 -- FzR/RConn1

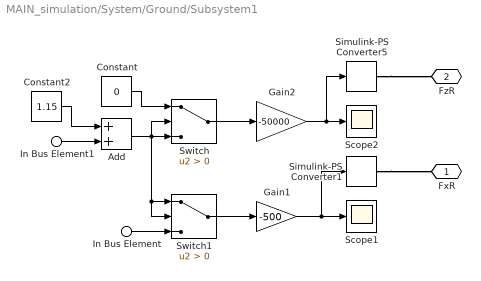
== system MAIN_simulation/System/Ground/Subsystem1 ==
  In Bus Element : Inport  PortName=SensorSignal  Element=Velocity.xAxis
  In Bus Element1 : Inport  PortName=SensorSignal  Element=Position.zAxis
  Add : Sum
  Constant : Constant  Value=0
  Constant2 : Constant  Value=1.15
  Gain1 : Gain  Gain=-500
  Gain2 : Gain  Gain=-50000
  Scope1 : Scope
  Scope2 : Scope
  Simulink-PS Converter1 : nesl_utility/Simulink-PS Converter  PhysicalDomain=network_engine_domain  SubClassName=ps_input  LeftPortType=input  RightPortType=output  PseudoPeriodic=off  Frequencies=[]  NoiseDistribution=none  NoiseParameters=[]  Unit=N  AffineConversion=off  FilteringAndDerivatives=filter  SimscapeFilterOrder=2  InputFilterTimeConstant=0.001  UdotUserProvided=0
      settings: SourceProductBaseCode=PW,SS
  Simulink-PS Converter5 : nesl_utility/Simulink-PS Converter  PhysicalDomain=network_engine_domain  SubClassName=ps_input  LeftPortType=input  RightPortType=output  PseudoPeriodic=off  Frequencies=[]  NoiseDistribution=none  NoiseParameters=[]  Unit=N  AffineConversion=off  FilteringAndDerivatives=filter  SimscapeFilterOrder=2  InputFilterTimeConstant=0.001  UdotUserProvided=0
      settings: SourceProductBaseCode=PW,SS
  Switch : Switch  Criteria=u2 > Threshold
  Switch1 : Switch  Criteria=u2 > Threshold
  FxR : PMIOPort  Side=Right
  FzR : PMIOPort  Port=2  Side=Right
  wires:
  Constant/1 -> Switch/1
  Gain2/1 -> Simulink-PS Converter5/1, Scope2/1
  In Bus Element1/1 -> Add/2
  Switch/1 -> Gain2/1
  Switch1/1 -> Gain1/1
  Constant2/1 -> Add/1
  In Bus Element/1 -> Switch1/3
  Gain1/1 -> Simulink-PS Converter1/1, Scope1/1
  Add/1 -> Switch1/2, Switch1/1, Switch/2, Switch/3
  connections:
  Simulink-PS Converter5/RConn1 -- FzR/RConn1
  Simulink-PS Converter1/RConn1 -- FxR/RConn1

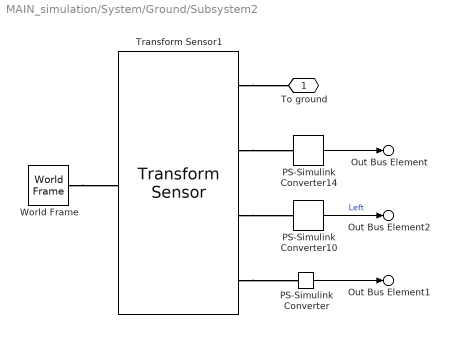
== system MAIN_simulation/System/Ground/Subsystem2 ==
  PS-Simulink Converter : nesl_utility/PS-Simulink Converter  PhysicalDomain=network_engine_domain  SubClassName=ps_output  LeftPortType=input  RightPortType=output  PseudoPeriodic=off  Frequencies=[]  Unit=inherit  AffineConversion=off
      settings: SourceProductBaseCode=PW,SS
  PS-Simulink Converter10 : nesl_utility/PS-Simulink Converter  PhysicalDomain=network_engine_domain  SubClassName=ps_output  LeftPortType=input  RightPortType=output  PseudoPeriodic=off  Frequencies=[]  Unit=inherit  AffineConversion=off
      settings: SourceProductBaseCode=PW,SS
  PS-Simulink Converter14 : nesl_utility/PS-Simulink Converter  PhysicalDomain=network_engine_domain  SubClassName=ps_output  LeftPortType=input  RightPortType=output  PseudoPeriodic=off  Frequencies=[]  Unit=inherit  AffineConversion=off
      settings: SourceProductBaseCode=PW,SS
  Transform Sensor1 : sm_lib/Frames and Transforms/Transform Sensor  MeasurementFrame=World  SenseAngle=off  SenseAxis=off  SenseAngle1=off  SenseAngle2=off  SenseAngle3=off  SenseQ=off  SenseR=off  SenseOmegaX=off  SenseOmegaY=off  SenseOmegaZ=off  SenseOmega1=off  SenseOmega2=off  SenseOmega3=off  SenseQDot=off  SenseRDot=off  SenseAlphaX=off  SenseAlphaY=off  SenseAlphaZ=off  SenseAlpha1=off  SenseAlpha2=off  SenseAlpha3=off  SenseQDDot=off  SenseRDDot=off  SenseX=on  SenseY=off  SenseZ=on  SenseRad=off  SenseAzim=off  SenseDist=off  SenseInc=off  SenseXDot=on  SenseYDot=off  SenseZDot=off  SenseRadDot=off  SenseAzimDot=off  SenseDistDot=off  SenseIncDot=off  SenseXDDot=off  SenseYDDot=off  SenseZDDot=off  SenseRadDDot=off  SenseAzimDDot=off  SenseDistDDot=off  SenseIncDDot=off
  World Frame : sm_lib/Frames and Transforms/World Frame
  To ground : PMIOPort  Side=Right
  Out Bus Element : Outport  PortName=SensorSignal  Element=Position.xAxis
  Out Bus Element2 : Outport  PortName=SensorSignal  Element=Position.zAxis
  Out Bus Element1 : Outport  PortName=SensorSignal  Element=Velocity.xAxis
  wires:
  PS-Simulink Converter/1 -> Out Bus Element1/1
  PS-Simulink Converter14/1 -> Out Bus Element/1
  PS-Simulink Converter10/1 -> Out Bus Element2/1  "Left"
  connections:
  World Frame/RConn1 -- Transform Sensor1/LConn1
  Transform Sensor1/RConn2 -- PS-Simulink Converter14/LConn1
  Transform Sensor1/RConn4 -- PS-Simulink Converter/LConn1
  Transform Sensor1/RConn3 -- PS-Simulink Converter10/LConn1
  Transform Sensor1/RConn1 -- To ground/RConn1

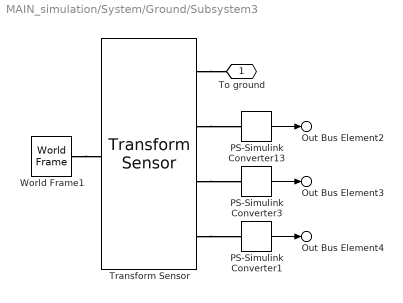
== system MAIN_simulation/System/Ground/Subsystem3 ==
  PS-Simulink Converter1 : nesl_utility/PS-Simulink Converter  PhysicalDomain=network_engine_domain  SubClassName=ps_output  LeftPortType=input  RightPortType=output  PseudoPeriodic=off  Frequencies=[]  Unit=inherit  AffineConversion=off
      settings: SourceProductBaseCode=PW,SS
  PS-Simulink Converter13 : nesl_utility/PS-Simulink Converter  PhysicalDomain=network_engine_domain  SubClassName=ps_output  LeftPortType=input  RightPortType=output  PseudoPeriodic=off  Frequencies=[]  Unit=inherit  AffineConversion=off
      settings: SourceProductBaseCode=PW,SS
  PS-Simulink Converter3 : nesl_utility/PS-Simulink Converter  PhysicalDomain=network_engine_domain  SubClassName=ps_output  LeftPortType=input  RightPortType=output  PseudoPeriodic=off  Frequencies=[]  Unit=inherit  AffineConversion=off
      settings: SourceProductBaseCode=PW,SS
  Transform Sensor : sm_lib/Frames and Transforms/Transform Sensor  MeasurementFrame=World  SenseAngle=off  SenseAxis=off  SenseAngle1=off  SenseAngle2=off  SenseAngle3=off  SenseQ=off  SenseR=off  SenseOmegaX=off  SenseOmegaY=off  SenseOmegaZ=off  SenseOmega1=off  SenseOmega2=off  SenseOmega3=off  SenseQDot=off  SenseRDot=off  SenseAlphaX=off  SenseAlphaY=off  SenseAlphaZ=off  SenseAlpha1=off  SenseAlpha2=off  SenseAlpha3=off  SenseQDDot=off  SenseRDDot=off  SenseX=on  SenseY=off  SenseZ=on  SenseRad=off  SenseAzim=off  SenseDist=off  SenseInc=off  SenseXDot=on  SenseYDot=off  SenseZDot=off  SenseRadDot=off  SenseAzimDot=off  SenseDistDot=off  SenseIncDot=off  SenseXDDot=off  SenseYDDot=off  SenseZDDot=off  SenseRadDDot=off  SenseAzimDDot=off  SenseDistDDot=off  SenseIncDDot=off
  World Frame1 : sm_lib/Frames and Transforms/World Frame
  To ground : PMIOPort  Side=Left
  Out Bus Element2 : Outport  PortName=SensorSignal  Element=Position.xAxis
  Out Bus Element3 : Outport  PortName=SensorSignal  Element=Position.zAxis
  Out Bus Element4 : Outport  PortName=SensorSignal  Element=Velocity.xAxis
  wires:
  PS-Simulink Converter1/1 -> Out Bus Element4/1
  PS-Simulink Converter13/1 -> Out Bus Element2/1
  PS-Simulink Converter3/1 -> Out Bus Element3/1
  connections:
  Transform Sensor/RConn2 -- PS-Simulink Converter13/LConn1
  Transform Sensor/RConn1 -- To ground/RConn1
  Transform Sensor/RConn3 -- PS-Simulink Converter3/LConn1
  World Frame1/RConn1 -- Transform Sensor/LConn1
  Transform Sensor/RConn4 -- PS-Simulink Converter1/LConn1

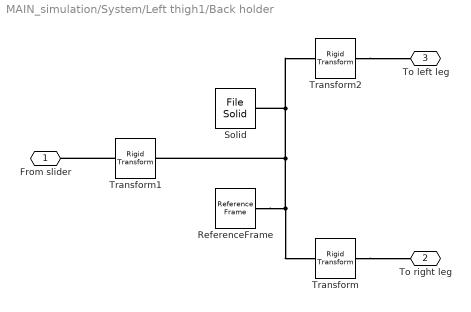
== system MAIN_simulation/System/Left thigh1/Back holder ==
  ReferenceFrame : sm_lib/Frames and Transforms/Reference Frame
  Solid : sm_lib/Body Elements/File Solid  ExtGeomFileName=Part1_Default_sldprt.STEP  UnitType=FromFile  ExtGeomFileUnits=m  StepReaderType=HEX  ExportConvexHullGeometry=off  InertiaType=Custom  Mass=40  MassUnits=kg  CenterOfMass=[0 0 0]  CenterOfMassUnits=mm  MomentsOfInertia=[0 0 0]  MomentsOfInertiaUnits=kg*mm^2  ProductsOfInertia=[0 0 0]  ProductsOfInertiaUnits=kg*mm^2  BasedOnType=Density  Density=1000  DensityUnits=kg/m^3  DoExposeReferenceFrame=on  SerializedFrames=<Frames/>  GraphicType=FromGeometry  MarkerShape=Sphere  MarkerSize=10  GraphicVisPropType=SimpleVisualProperties  GraphicDiffuseColor=smiData.Solid(3).color  GraphicSpecularColor=[0.5 0.5 0.5 1.0]  GraphicAmbientColor=[0.15 0.15 0.15 1.0]  GraphicEmissiveColor=[0.0 0.0 0.0 1.0]  GraphicShininess=75  GraphicOpacity=smiData.Solid(3).opacity
  Transform : sm_lib/Frames and Transforms/Rigid Transform  TranslationMethod=Cartesian  TranslationStandardOffset=0  TranslationLengthUnit=mm  TranslationStandardAxis=+Z  TranslationCartesianOffset=smiData.RigidTransform(9).translation  TranslationROffset=0  TranslationROffsetUnits=m  TranslationZOffset=0  TranslationZOffsetUnits=m  TranslationThetaOffset=0  TranslationThetaOffsetUnits=deg  RotationMethod=ArbitraryAxis  RotationAngleUnits=rad  RotationStandardAxis=+Z  RotationAngle=smiData.RigidTransform(9).angle  RotationArbitraryAxis=smiData.RigidTransform(9).axis  FollAlignAxisA=+X  BaseAlignAxisA=+Y  FollAlignAxisB=+Y  BaseAlignAxisB=+Z  RotationSequenceAxes=FollowerAxes  RotationSequence=XYX  RotationSequenceAngles=[0 0 0]  RotationSequenceAnglesUnits=deg  RotationMatrix=[1 0 0; 0 1 0; 0 0 1]
  Transform1 : sm_lib/Frames and Transforms/Rigid Transform  TranslationMethod=Cartesian  TranslationStandardOffset=0  TranslationLengthUnit=mm  TranslationStandardAxis=+Z  TranslationCartesianOffset=smiData.RigidTransform(11).translation  TranslationROffset=0  TranslationROffsetUnits=m  TranslationZOffset=0  TranslationZOffsetUnits=m  TranslationThetaOffset=0  TranslationThetaOffsetUnits=deg  RotationMethod=ArbitraryAxis  RotationAngleUnits=rad  RotationStandardAxis=+Z  RotationAngle=smiData.RigidTransform(11).angle  RotationArbitraryAxis=smiData.RigidTransform(11).axis  FollAlignAxisA=+X  BaseAlignAxisA=+Y  FollAlignAxisB=+Y  BaseAlignAxisB=+Z  RotationSequenceAxes=FollowerAxes  RotationSequence=XYX  RotationSequenceAngles=[0 0 0]  RotationSequenceAnglesUnits=deg  RotationMatrix=[1 0 0; 0 1 0; 0 0 1]
  Transform2 : sm_lib/Frames and Transforms/Rigid Transform  TranslationMethod=Cartesian  TranslationStandardOffset=0  TranslationLengthUnit=mm  TranslationStandardAxis=+Z  TranslationCartesianOffset=smiData.RigidTransform(13).translation  TranslationROffset=0  TranslationROffsetUnits=m  TranslationZOffset=0  TranslationZOffsetUnits=m  TranslationThetaOffset=0  TranslationThetaOffsetUnits=deg  RotationMethod=ArbitraryAxis  RotationAngleUnits=rad  RotationStandardAxis=+Z  RotationAngle=smiData.RigidTransform(13).angle  RotationArbitraryAxis=smiData.RigidTransform(13).axis  FollAlignAxisA=+X  BaseAlignAxisA=+Y  FollAlignAxisB=+Y  BaseAlignAxisB=+Z  RotationSequenceAxes=FollowerAxes  RotationSequence=XYX  RotationSequenceAngles=[0 0 0]  RotationSequenceAnglesUnits=deg  RotationMatrix=[1 0 0; 0 1 0; 0 0 1]
  From slider : PMIOPort  Side=Left
  To right leg : PMIOPort  Port=2  Side=Right
  To left leg : PMIOPort  Port=3  Side=Right
  connections:
  Solid/RConn1 -- Transform2/LConn1 -- ReferenceFrame/RConn1 -- Transform/LConn1 -- Transform1/LConn1
  Transform/RConn1 -- To right leg/RConn1
  Transform1/RConn1 -- From slider/RConn1
  Transform2/RConn1 -- To left leg/RConn1

== system MAIN_simulation/System/Left thigh1/Base_1_RIGID ==
  ReferenceFrame : sm_lib/Frames and Transforms/Reference Frame
  Solid : sm_lib/Body Elements/File Solid  ExtGeomFileName=Base_Default_sldprt.STEP  UnitType=FromFile  ExtGeomFileUnits=m  StepReaderType=HEX  ExportConvexHullGeometry=off  InertiaType=Custom  Mass=smiData.Solid(6).mass  MassUnits=kg  CenterOfMass=smiData.Solid(6).CoM  CenterOfMassUnits=mm  MomentsOfInertia=smiData.Solid(6).MoI  MomentsOfInertiaUnits=kg*mm^2  ProductsOfInertia=smiData.Solid(6).PoI  ProductsOfInertiaUnits=kg*mm^2  BasedOnType=Density  Density=1000  DensityUnits=kg/m^3  DoExposeReferenceFrame=on  SerializedFrames=<Frames/>  GraphicType=FromGeometry  MarkerShape=Sphere  MarkerSize=10  GraphicVisPropType=SimpleVisualProperties  GraphicDiffuseColor=smiData.Solid(6).color  GraphicSpecularColor=[0.5 0.5 0.5 1.0]  GraphicAmbientColor=[0.15 0.15 0.15 1.0]  GraphicEmissiveColor=[0.0 0.0 0.0 1.0]  GraphicShininess=75  GraphicOpacity=smiData.Solid(6).opacity
  Transform : sm_lib/Frames and Transforms/Rigid Transform  TranslationMethod=Cartesian  TranslationStandardOffset=0  TranslationLengthUnit=mm  TranslationStandardAxis=+Z  TranslationCartesianOffset=smiData.RigidTransform(1).translation  TranslationROffset=0  TranslationROffsetUnits=m  TranslationZOffset=0  TranslationZOffsetUnits=m  TranslationThetaOffset=0  TranslationThetaOffsetUnits=deg  RotationMethod=ArbitraryAxis  RotationAngleUnits=rad  RotationStandardAxis=+Z  RotationAngle=smiData.RigidTransform(1).angle  RotationArbitraryAxis=smiData.RigidTransform(1).axis  FollAlignAxisA=+X  BaseAlignAxisA=+Y  FollAlignAxisB=+Y  BaseAlignAxisB=+Z  RotationSequenceAxes=FollowerAxes  RotationSequence=XYX  RotationSequenceAngles=[0 0 0]  RotationSequenceAnglesUnits=deg  RotationMatrix=[1 0 0; 0 1 0; 0 0 1]
  Transform1 : sm_lib/Frames and Transforms/Rigid Transform  TranslationMethod=Cartesian  TranslationStandardOffset=0  TranslationLengthUnit=mm  TranslationStandardAxis=+Z  TranslationCartesianOffset=smiData.RigidTransform(3).translation  TranslationROffset=0  TranslationROffsetUnits=m  TranslationZOffset=0  TranslationZOffsetUnits=m  TranslationThetaOffset=0  TranslationThetaOffsetUnits=deg  RotationMethod=ArbitraryAxis  RotationAngleUnits=rad  RotationStandardAxis=+Z  RotationAngle=smiData.RigidTransform(3).angle  RotationArbitraryAxis=smiData.RigidTransform(3).axis  FollAlignAxisA=+X  BaseAlignAxisA=+Y  FollAlignAxisB=+Y  BaseAlignAxisB=+Z  RotationSequenceAxes=FollowerAxes  RotationSequence=XYX  RotationSequenceAngles=[0 0 0]  RotationSequenceAnglesUnits=deg  RotationMatrix=[1 0 0; 0 1 0; 0 0 1]
  From world frame : PMIOPort  Side=Left
  To slider : PMIOPort  Port=2  Side=Right
  connections:
  Solid/RConn1 -- Transform/LConn1 -- ReferenceFrame/RConn1 -- Transform1/LConn1
  Transform/RConn1 -- To slider/RConn1
  Transform1/RConn1 -- From world frame/RConn1
